simulink model "w3_3"  (R2020b)
settings: Solver=VariableStepAuto  StartTime=0.0  StopTime=10.0  RelTol=1e-3
model workspace (MAT data in the model file):
  I = 5
  Kf = 1
  Ki = 0.0723
  Kp = 0.0614
  PBmax = 1500
  Rr = 1.25
  TB = 0.01
  ctrl = 1
  g = 32.18
  m = 50
  mu = [0 0.4 0.8 0.97 1 0.98 0.96 0.94 0.92 0.9 0.88 0.855 0.83 0.81 0.79 0.77 0.75 0.73 0.72 0.71 0.7]
  slip = [0 0.05 0.1 0.15 0.2 0.25 0.3 0.35 0.4 0.45 0.5 0.55 0.6 0.65 0.7 0.75 0.8 0.85 0.9 0.95 1]
  v0 = 88
settings Model: Creator=MY lenovo  LastModifiedBy=MY lenovo

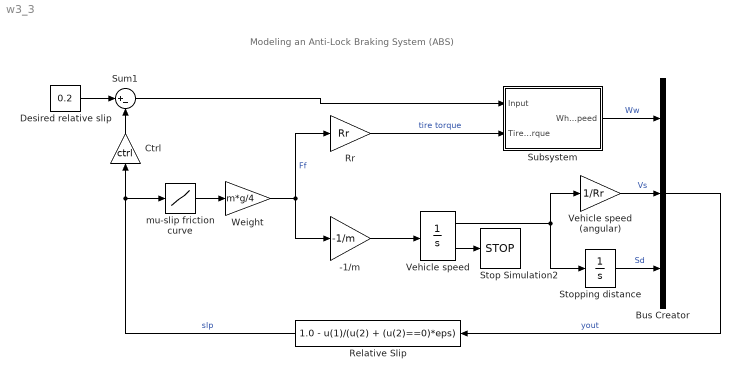
== system w3_3 ==
  note: Modeling an Anti-Lock Braking System (ABS)
  -1/m : Gain  Gain=-1/m  SaturateOnIntegerOverflow=on  OutDataTypeStr=Inherit: Same as input  ParamDataTypeStr=Inherit: Same as input
  Bus Creator : BusCreator  Inputs=3
  Ctrl : Gain  Gain=ctrl  SaturateOnIntegerOverflow=on  OutDataTypeStr=Inherit: Same as input  ParamDataTypeStr=Inherit: Same as input
  Desired relative slip : Constant  Value=0.2
  Relative Slip : Fcn  Expr=1.0 - u(1)/(u(2) + (u(2)==0)*eps)
  Rr : Gain  Gain=Rr  SaturateOnIntegerOverflow=on  OutDataTypeStr=Inherit: Same as input  ParamDataTypeStr=Inherit: Same as input
  Stop Simulation2 : Stop
  Stopping distance : Integrator  UpperSaturationLimit=1000  LowerSaturationLimit=0
  Subsystem : Subsystem
  Sum1 : Sum  Inputs=|+-  InputSameDT=on  SaturateOnIntegerOverflow=on  OutDataTypeStr=Inherit: Same as first input
  Vehicle speed : Integrator  InitialCondition=v0  LimitOutput=on  UpperSaturationLimit=1000  LowerSaturationLimit=0  ShowSaturationPort=on
  Vehicle speed (angular) : Gain  Gain=1/Rr  SaturateOnIntegerOverflow=on  OutDataTypeStr=Inherit: Same as input  ParamDataTypeStr=Inherit: Same as input
  Weight : Gain  Gain=m*g/4  SaturateOnIntegerOverflow=on  OutDataTypeStr=Inherit: Same as input  ParamDataTypeStr=Inherit: Same as input
  mu-slip friction curve : Lookup_n-D  NumberOfTableDimensions=1  BreakpointsForDimension1=slip  Table=mu  SaturateOnIntegerOverflow=on  InputSameDT=on
  wires:
  Rr/1 -> Subsystem/2(Tire Torque)  "tire torque"
  Subsystem/1(WheelSpeed) -> Bus Creator/1  "Ww"
  Ctrl/1 -> Sum1/2
  Vehicle speed/2 -> Stop Simulation2/1
  Weight/1 -> -1/m/1, Rr/1  "Ff"
  -1/m/1 -> Vehicle speed/1
  Desired relative slip/1 -> Sum1/1
  mu-slip friction curve/1 -> Weight/1
  Vehicle speed/1 -> Stopping distance/1, Vehicle speed (angular)/1
  Vehicle speed (angular)/1 -> Bus Creator/2  "Vs"
  Relative Slip/1 -> mu-slip friction curve/1, Ctrl/1  "slp"
  Bus Creator/1 -> Relative Slip/1  "yout"
  Stopping distance/1 -> Bus Creator/3  "Sd"
  Sum1/1 -> Subsystem/1(Input)

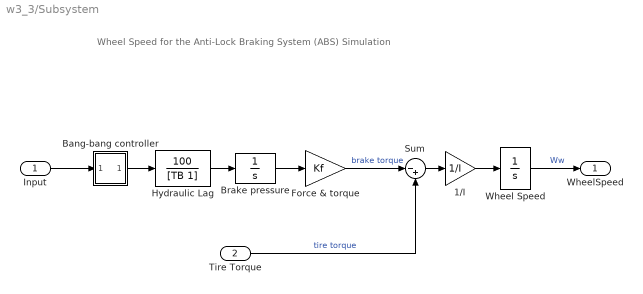
== system w3_3/Subsystem ==
  note: Wheel Speed for the
      | Anti-Lock Braking System (ABS) Simulation
  Input : Inport  SampleTime=0
  Tire Torque : Inport  Port=2
  1/I : Gain  Gain=1/I  SaturateOnIntegerOverflow=on  OutDataTypeStr=Inherit: Same as input  ParamDataTypeStr=Inherit: Same as input
  Bang-bang controller : Subsystem  mask(Sign){}
      mask help: y = sign(x)
      mask Help: Sign Function:\n\t\t\ty = 1 if x > 0\n\t\t\ty = 0 if x = 0\n\t\t\ty = -1 if x < 0
      mask Display: plot(-50,-50,50,50,[-50,50],[0,0],[0,0],[-50,50],[-40,0],[-30,-30],[0,40],[30,30])
  Brake pressure : Integrator  LimitOutput=on  UpperSaturationLimit=PBmax  LowerSaturationLimit=0
  Force & torque : Gain  Gain=Kf  SaturateOnIntegerOverflow=on  OutDataTypeStr=Inherit: Same as input  ParamDataTypeStr=Inherit: Same as input
  "Hydraulic Lag " : TransferFcn  Numerator=[100]  Denominator=[TB 1]
  Sum : Sum  Inputs=|-+  InputSameDT=on  SaturateOnIntegerOverflow=on  OutDataTypeStr=Inherit: Same as first input
  Wheel Speed : Integrator  InitialCondition=v0/Rr  LimitOutput=on  UpperSaturationLimit=1000  LowerSaturationLimit=0
  WheelSpeed : Outport  VectorParamsAs1DForOutWhenUnconnected=off
  wires:
  Input/1 -> Bang-bang controller/1(in_1)
  "Hydraulic Lag "/1 -> Brake pressure/1
  Force & torque/1 -> Sum/1  "brake torque"
  Tire Torque/1 -> Sum/2  "tire torque"
  Brake pressure/1 -> Force & torque/1
  Bang-bang controller/1(out_1) -> "Hydraulic Lag "/1
  Sum/1 -> 1/I/1
  1/I/1 -> Wheel Speed/1
  Wheel Speed/1 -> WheelSpeed/1  "Ww"

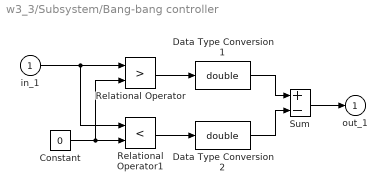
== system w3_3/Subsystem/Bang-bang controller ==
  in_1 : Inport
  Constant : Constant  Value=0
  Data Type Conversion1 : DataTypeConversion  OutDataTypeStr=double  SaturateOnIntegerOverflow=on  RndMeth=Zero
  Data Type Conversion2 : DataTypeConversion  OutDataTypeStr=double  SaturateOnIntegerOverflow=on  RndMeth=Zero
  Relational Operator : RelationalOperator  Operator=>  OutDataTypeStr=boolean  RndMeth=Nearest  InputSameDT=on
  Relational Operator1 : RelationalOperator  Operator=<  OutDataTypeStr=boolean  RndMeth=Nearest  InputSameDT=on
  Sum : Sum  Inputs=+-  InputSameDT=on  SaturateOnIntegerOverflow=on  OutDataTypeStr=Inherit: Same as first input
  out_1 : Outport  InitialOutput=0  VectorParamsAs1DForOutWhenUnconnected=off
  wires:
  Data Type Conversion2/1 -> Sum/2
  Data Type Conversion1/1 -> Sum/1
  Sum/1 -> out_1/1
  Relational Operator/1 -> Data Type Conversion1/1
  Relational Operator1/1 -> Data Type Conversion2/1
  Constant/1 -> Relational Operator/2, Relational Operator1/2
  in_1/1 -> Relational Operator1/1, Relational Operator/1
